simulink subsystem "Estimator"  (R2022a)
settings: Solver=VariableStepAuto  StartTime=0.0  StopTime=10.0  RelTol=1e-3
values from neighbouring files (symbols this model uses):
  C = eye(3)    [DAE_Circuit_main.m]
undefined symbols (not defined in the file or in its folder): C_1, C_4, R_1, R_2, R_3, R_4, x_0_2D
settings Model: Creator=tyevans  LastModifiedBy=tyevans

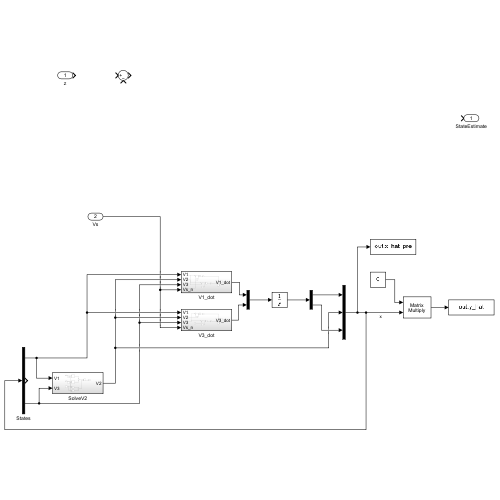
[thumbnail: Simulink's stored preview of the top-level diagram]
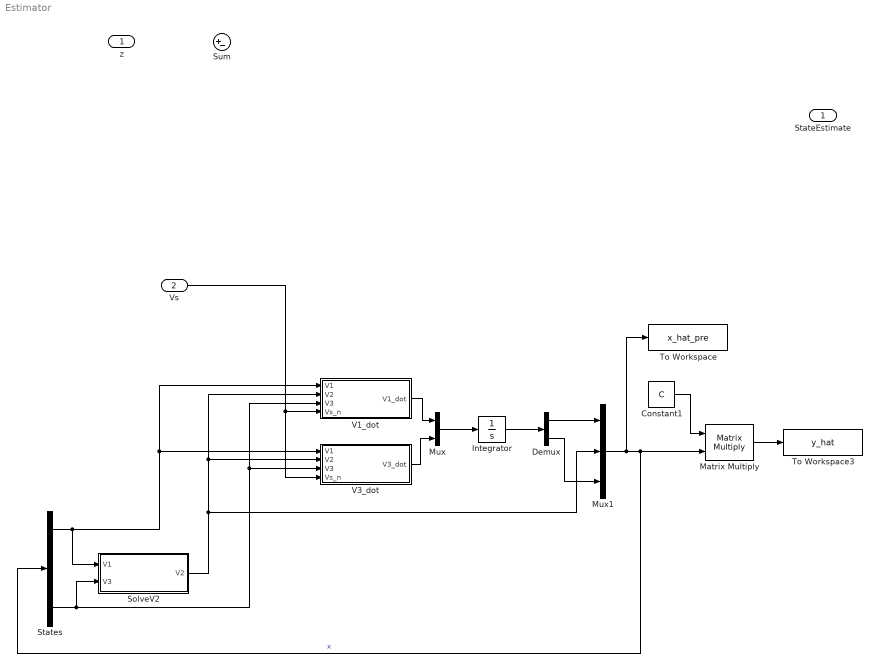
== system Estimator ==
  z : Inport
  Vs : Inport  Port=2
  Constant1 : Constant  Value=C  VectorParams1D=off
  Demux : Demux  Outputs=2
  Integrator : Integrator  InitialCondition=x_0_2D
  Matrix Multiply : Product  Multiplication=Matrix(*)
  Mux : Mux  Inputs=2
  Mux1 : Mux  Inputs=3
  SolveV2 : Subsystem
  States : Demux  Outputs=3
  Sum : Sum  Inputs=|+-
  To Workspace : ToWorkspace  VariableName=x_hat_pre  SampleTime=-1
  To Workspace3 : ToWorkspace  VariableName=y_hat  SampleTime=-1
  V1_dot : Subsystem
  V3_dot : Subsystem
  StateEstimate : Outport
  wires:
  Mux1/1 -> To Workspace/1, Matrix Multiply/2, States/1  "x"
  States/1 -> SolveV2/1(V1), V1_dot/1(V1), V3_dot/1(V1)
  Mux/1 -> Integrator/1
  Vs/1 -> V1_dot/4(Vs_n), V3_dot/4(Vs_n)
  V3_dot/1(V3_dot) -> Mux/2
  Demux/1 -> Mux1/1
  V1_dot/1(V1_dot) -> Mux/1
  Demux/2 -> Mux1/3
  Constant1/1 -> Matrix Multiply/1
  Integrator/1 -> Demux/1
  Matrix Multiply/1 -> To Workspace3/1
  SolveV2/1(V2) -> Mux1/2, V3_dot/2(V2), V1_dot/2(V2)
  States/3 -> V3_dot/3(V3), V1_dot/3(V3), SolveV2/2(V3)

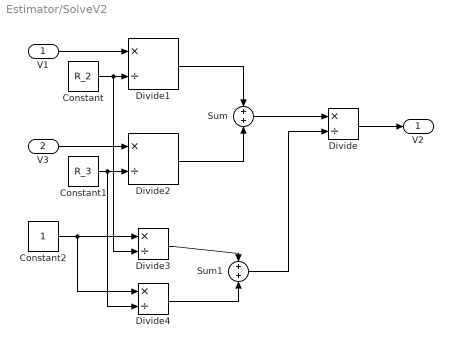
== system Estimator/SolveV2 ==
  V1 : Inport
  V3 : Inport  Port=2
  Constant : Constant  Value=R_2
  Constant1 : Constant  Value=R_3
  Constant2 : Constant
  Divide{,1..4} (5 alike) : Product  Inputs=*/
  Sum : Sum
  Sum1 : Sum
  V2 : Outport
  wires:
  V1/1 -> Divide1/1
  Constant/1 -> Divide3/2, Divide1/2
  Constant1/1 -> Divide4/2, Divide2/2
  V3/1 -> Divide2/1
  Divide1/1 -> Sum/1
  Divide2/1 -> Sum/2
  Sum/1 -> Divide/1
  Divide/1 -> V2/1
  Constant2/1 -> Divide4/1, Divide3/1
  Divide3/1 -> Sum1/1
  Divide4/1 -> Sum1/2
  Sum1/1 -> Divide/2

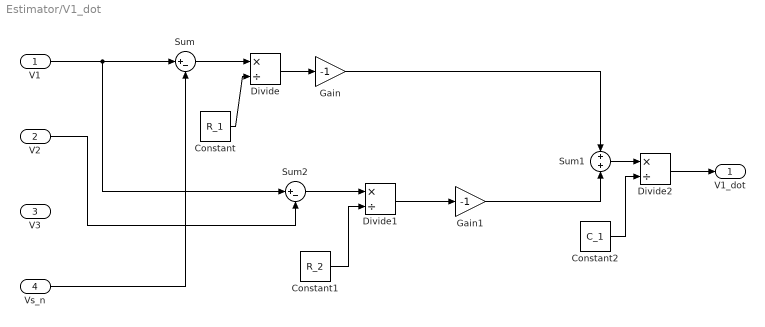
== system Estimator/V1_dot ==
  V1 : Inport
  V2 : Inport  Port=2
  V3 : Inport  Port=3
  Vs_n : Inport  Port=4
  Constant : Constant  Value=R_1
  Constant1 : Constant  Value=R_2
  Constant2 : Constant  Value=C_1
  Divide : Product  Inputs=*/
  Divide1 : Product  Inputs=*/
  Divide2 : Product  Inputs=*/
  Gain : Gain  Gain=-1
  Gain1 : Gain  Gain=-1
  Sum : Sum  Inputs=|+-
  Sum1 : Sum
  Sum2 : Sum  Inputs=|+-
  V1_dot : Outport
  wires:
  V1/1 -> Sum2/1, Sum/1
  Vs_n/1 -> Sum/2
  Sum/1 -> Divide/1
  Constant/1 -> Divide/2
  Divide/1 -> Gain/1
  Gain/1 -> Sum1/1
  V2/1 -> Sum2/2
  Sum2/1 -> Divide1/1
  Constant1/1 -> Divide1/2
  Divide2/1 -> V1_dot/1
  Sum1/1 -> Divide2/1
  Divide1/1 -> Gain1/1
  Gain1/1 -> Sum1/2
  Constant2/1 -> Divide2/2

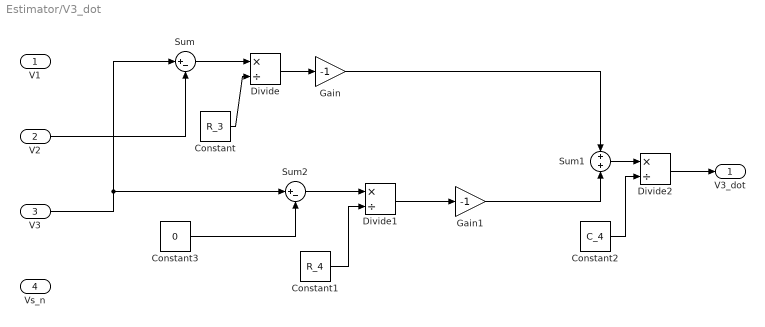
== system Estimator/V3_dot ==
  V1 : Inport
  V2 : Inport  Port=2
  V3 : Inport  Port=3
  Vs_n : Inport  Port=4
  Constant : Constant  Value=R_3
  Constant1 : Constant  Value=R_4
  Constant2 : Constant  Value=C_4
  Constant3 : Constant  Value=0
  Divide : Product  Inputs=*/
  Divide1 : Product  Inputs=*/
  Divide2 : Product  Inputs=*/
  Gain : Gain  Gain=-1
  Gain1 : Gain  Gain=-1
  Sum : Sum  Inputs=|+-
  Sum1 : Sum
  Sum2 : Sum  Inputs=|+-
  V3_dot : Outport
  wires:
  Sum/1 -> Divide/1
  Constant/1 -> Divide/2
  Divide/1 -> Gain/1
  Gain/1 -> Sum1/1
  Sum2/1 -> Divide1/1
  Constant1/1 -> Divide1/2
  Divide2/1 -> V3_dot/1
  Sum1/1 -> Divide2/1
  Divide1/1 -> Gain1/1
  Gain1/1 -> Sum1/2
  Constant2/1 -> Divide2/2
  V3/1 -> Sum2/1, Sum/1
  V2/1 -> Sum/2
  Constant3/1 -> Sum2/2
